simulink model "PMAFPLL"  (R2020b)
settings: Solver=VariableStepAuto  StartTime=0.0  StopTime=10.0  FixedStep=Ts  RelTol=1e-3
values from neighbouring files (symbols this model uses):
  N = T_MAF/Ts    (= 200)    [maf_filter.m]
undefined symbols (not defined in the file or in its folder): A_frq_step, A_phase_step, f_rad, ki, kp, t_frq_step, t_phase_step, V_g, var_noise
libraries: simulink x6, bach_library x4
settings Model: Creator=Kasper Laustsen  LastModifiedBy=Kasper Laustsen

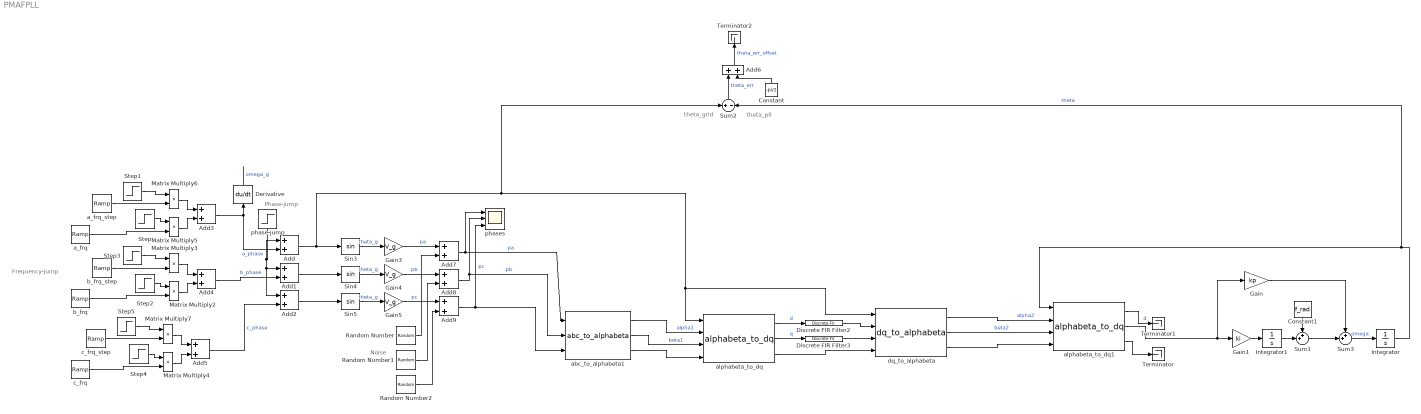
== system PMAFPLL ==
  note: Frequency-jump
  note: Noise
  note: Phase-jump
  note: theta_grid
  note: theta_pll
  Add{,1..9} (10 alike) : Sum
  Constant : Constant  Value=-pi/2
  Constant1 : Constant  Value=f_rad
  Derivative : Derivative
  Discrete FIR Filter2 : DiscreteFir  Coefficients=[ones(1,N).*1/N]
  Discrete FIR Filter3 : DiscreteFir  Coefficients=[ones(1,N).*1/N]
  Gain : Gain  Gain=kp
  Gain1 : Gain  Gain=ki
  Gain3 : Gain  Gain=V_g
  Gain4 : Gain  Gain=V_g
  Gain5 : Gain  Gain=V_g
  Integrator : Integrator
  Integrator1 : Integrator
  Matrix Multiply{2..7} (6 alike) : Product
  Random Number : RandomNumber  Variance=var_noise
  Random Number1 : RandomNumber  Variance=var_noise  Seed=1
  Random Number2 : RandomNumber  Variance=var_noise  Seed=2
  Sin3 : Trigonometry
  Sin4 : Trigonometry
  Sin5 : Trigonometry
  Step : Step  Time=t_frq_step  Before=1  After=0  SampleTime=0
  Step1 : Step  Time=t_frq_step  SampleTime=0
  Step2 : Step  Time=t_frq_step  Before=1  After=0  SampleTime=0
  Step3 : Step  Time=t_frq_step  SampleTime=0
  Step4 : Step  Time=t_frq_step  Before=1  After=0  SampleTime=0
  Step5 : Step  Time=t_frq_step  SampleTime=0
  Sum1 : Sum  Inputs=++|
  Sum2 : Sum  Inputs=+|-
  Sum3 : Sum  Inputs=++|
  Terminator : Terminator
  Terminator1 : Terminator
  Terminator2 : Terminator
  a_frq : simulink/Sources/Ramp  slope=f_rad  start=0  InitialOutput=0
  a_frq_step : simulink/Sources/Ramp  slope=f_rad*A_frq_step  start=t_frq_step  InitialOutput=t_frq_step*f_rad
  abc_to_alphabeta1 : bach_library/abc_to_alphabeta  SystemSampleTime=-1  VariantActivationTime=update diagram  Latency=0  AutoFrameSizeCalculation=off
  alphabeta_to_dq : bach_library/alphabeta_to_dq  SystemSampleTime=-1  VariantActivationTime=update diagram  Latency=0  AutoFrameSizeCalculation=off
  alphabeta_to_dq1 : bach_library/alphabeta_to_dq  SystemSampleTime=-1  VariantActivationTime=update diagram  Latency=0  AutoFrameSizeCalculation=off
  b_frq : simulink/Sources/Ramp  slope=f_rad  start=0  InitialOutput=f_rad/3
  b_frq_step : simulink/Sources/Ramp  slope=f_rad*A_frq_step  start=t_frq_step  InitialOutput=t_frq_step*f_rad+f_rad/3
  c_frq : simulink/Sources/Ramp  slope=f_rad  start=0  InitialOutput=f_rad*2/3
  c_frq_step : simulink/Sources/Ramp  slope=f_rad*A_frq_step  start=t_frq_step  InitialOutput=t_frq_step*f_rad+f_rad*2/3
  dq_to_alphabeta : bach_library/dq_to_alphabeta  SystemSampleTime=-1  VariantActivationTime=update diagram  Latency=0  AutoFrameSizeCalculation=off
  phase-jump : Step  Time=t_phase_step  After=A_phase_step  SampleTime=0
  phases : Scope  NumInputPorts=3
  wires:
  Add4/1 -> Add1/2  "b_phase"
  Random Number1/1 -> Add8/2
  Add3/1 -> Add/2, Derivative/1  "a_phase"
  Add9/1 -> abc_to_alphabeta1/3, phases/3  "pc"
  Derivative/1 -> ?  "omega_g"
  Gain5/1 -> Add9/1  "pc"
  b_frq_step/1 -> Matrix Multiply3/2
  Matrix Multiply4/1 -> Add5/2
  Matrix Multiply6/1 -> Add3/1
  Sin4/1 -> Gain4/1  "theta_g"
  b_frq/1 -> Matrix Multiply2/2
  Matrix Multiply3/1 -> Add4/1
  c_frq_step/1 -> Matrix Multiply7/2
  Step5/1 -> Matrix Multiply7/1
  Matrix Multiply2/1 -> Add4/2
  Step4/1 -> Matrix Multiply4/1
  Add8/1 -> phases/2, abc_to_alphabeta1/2  "pb"
  Add7/1 -> abc_to_alphabeta1/1, phases/1  "pa"
  a_frq_step/1 -> Matrix Multiply6/2
  Step2/1 -> Matrix Multiply2/1
  Add1/1 -> Sin4/1
  Random Number/1 -> Add7/2
  phase-jump/1 -> Add/1, Add2/1, Add1/1
  c_frq/1 -> Matrix Multiply4/2
  Add2/1 -> Sin5/1
  Random Number2/1 -> Add9/2
  Sin5/1 -> Gain5/1  "theta_g"
  Sin3/1 -> Gain3/1  "theta_g"
  Step1/1 -> Matrix Multiply6/1
  Add5/1 -> Add2/2  "c_phase"
  Gain3/1 -> Add7/1  "pa"
  Step3/1 -> Matrix Multiply3/1
  Matrix Multiply7/1 -> Add5/1
  Step/1 -> Matrix Multiply5/1
  a_frq/1 -> Matrix Multiply5/2
  Matrix Multiply5/1 -> Add3/2
  Gain4/1 -> Add8/1  "pb"
  Constant1/1 -> Sum1/1
  Sum1/1 -> Sum3/2
  Sum3/1 -> Integrator/1  "omega"
  Gain1/1 -> Integrator1/1
  Gain/1 -> Sum3/1
  alphabeta_to_dq1/2 -> Gain1/1, Gain/1
  Integrator1/1 -> Sum1/2
  abc_to_alphabeta1/1 -> alphabeta_to_dq/2  "alpha1"
  abc_to_alphabeta1/2 -> alphabeta_to_dq/3  "beta1"
  abc_to_alphabeta1/3 -> alphabeta_to_dq/4
  alphabeta_to_dq/3 -> dq_to_alphabeta/4
  alphabeta_to_dq/1 -> Discrete FIR Filter2/1  "d"
  alphabeta_to_dq/2 -> Discrete FIR Filter3/1  "q"
  Discrete FIR Filter3/1 -> dq_to_alphabeta/3
  Discrete FIR Filter2/1 -> dq_to_alphabeta/2
  dq_to_alphabeta/1 -> alphabeta_to_dq1/2  "alpha2"
  dq_to_alphabeta/2 -> alphabeta_to_dq1/3  "beta2"
  dq_to_alphabeta/3 -> alphabeta_to_dq1/4
  alphabeta_to_dq1/3 -> Terminator/1
  alphabeta_to_dq1/1 -> Terminator1/1  "d"
  Add6/1 -> Terminator2/1  "theta_err_offset"
  Integrator/1 -> Sum2/2, alphabeta_to_dq1/1  "theta"
  Add/1 -> Sum2/1, dq_to_alphabeta/1, alphabeta_to_dq/1, Sin3/1
  Sum2/1 -> Add6/1  "theta_err"
  Constant/1 -> Add6/2
